simulink model "L21MSDsim"  (R2020a)
settings: Solver=FixedStepAuto  StartTime=0.0  StopTime=10  FixedStep=0.001  RelTol=1e-3
InitFcn:
  | L21MSDparameters;
values from neighbouring files (symbols this model uses):
  A = [0 1 ; -k/m -b/m]    [L21MSDparameters.m]
  B = [0 ; 1/m]    [L21MSDparameters.m]
  C = [1 0]    [L21MSDparameters.m]
  L = place(A',C',[-10 -20])'    [L21MSDparameters.m]
  x0 = [1; 0.5]    [L21MSDparameters.m]
  x0hat = [x0(1); 0]    [L21MSDparameters.m]
undefined symbols (not defined in the file or in its folder): LKB
libraries: simulink x1
settings Model: Creator=vcichella  LastModifiedBy=vcichella

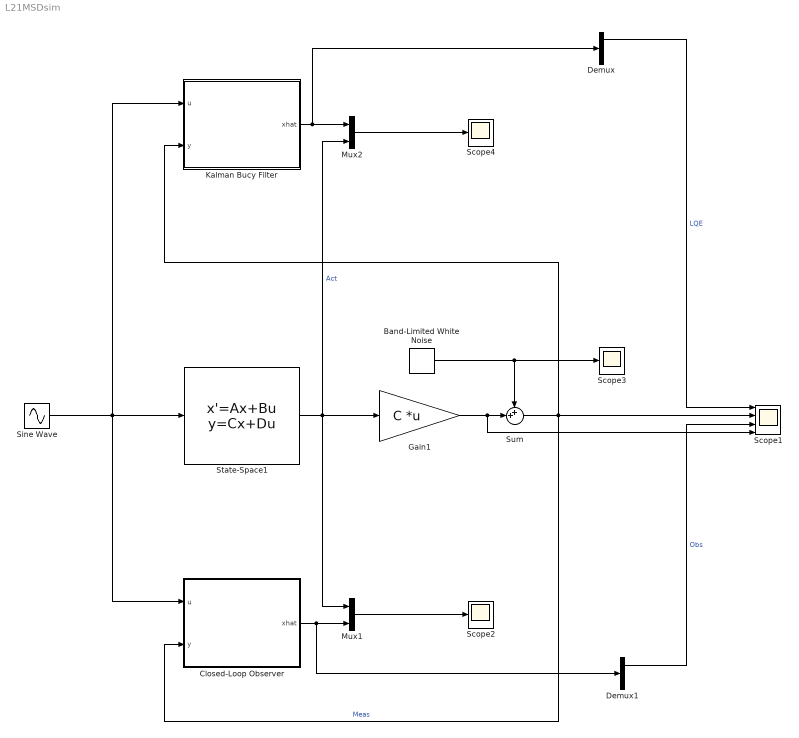
== system L21MSDsim ==
  Band-Limited White Noise : simulink/Sources/Band-Limited White Noise  Cov=[0.01]  Ts=0.01  seed=[23341]
  Closed-Loop Observer : Subsystem
  Demux : Demux  Outputs=2
  Demux1 : Demux  Outputs=2
  Gain1 : Gain  Gain=C  Multiplication=Matrix(K*u)
  Kalman Bucy Filter : Subsystem
  Mux1 : Mux  Inputs=2
  Mux2 : Mux  Inputs=2
  Scope1 : Scope  NumInputPorts=4
  Scope2 : Scope
  Scope3 : Scope
  Scope4 : Scope
  Sine Wave : Sin  Frequency=0.1  SampleTime=0
  State-Space1 : StateSpace  A=A  B=B  C=eye(size(A))  D=zeros(2,1)  InitialCondition=x0
  Sum : Sum  Inputs=++|
  wires:
  State-Space1/1 -> Mux2/2, Mux1/1, Gain1/1  "Act"
  Sine Wave/1 -> Kalman Bucy Filter/1(u), Closed-Loop Observer/1(u), State-Space1/1
  Closed-Loop Observer/1(xhat) -> Mux1/2, Demux1/1
  Mux1/1 -> Scope2/1
  Sum/1 -> Kalman Bucy Filter/2(y), Scope1/2, Closed-Loop Observer/2(y)  "Meas"
  Gain1/1 -> Scope1/4, Sum/2
  Band-Limited White Noise/1 -> Sum/1, Scope3/1
  Mux2/1 -> Scope4/1
  Kalman Bucy Filter/1(xhat) -> Mux2/1, Demux/1
  Demux1/1 -> Scope1/3  "Obs"
  Demux/1 -> Scope1/1  "LQE"

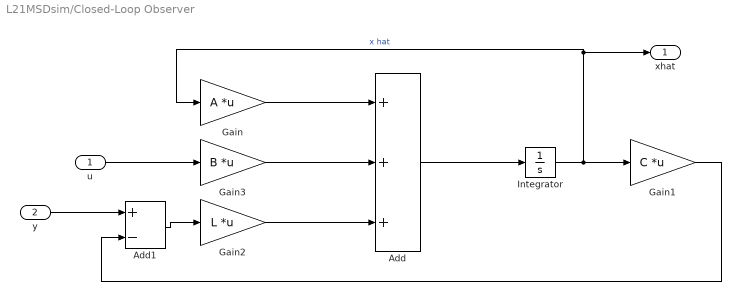
== system L21MSDsim/Closed-Loop Observer ==
  u : Inport
  y : Inport  Port=2
  Add : Sum  Inputs=+++
  Add1 : Sum  Inputs=+-
  Gain : Gain  Gain=A  Multiplication=Matrix(K*u)
  Gain1 : Gain  Gain=C  Multiplication=Matrix(K*u)
  Gain2 : Gain  Gain=L  Multiplication=Matrix(K*u)
  Gain3 : Gain  Gain=B  Multiplication=Matrix(K*u)
  Integrator : Integrator  InitialCondition=x0hat
  xhat : Outport
  wires:
  Integrator/1 -> xhat/1, Gain/1, Gain1/1  "x hat"
  Add/1 -> Integrator/1
  Gain/1 -> Add/1
  Gain1/1 -> Add1/2
  Add1/1 -> Gain2/1
  y/1 -> Add1/1
  Gain2/1 -> Add/3
  u/1 -> Gain3/1
  Gain3/1 -> Add/2

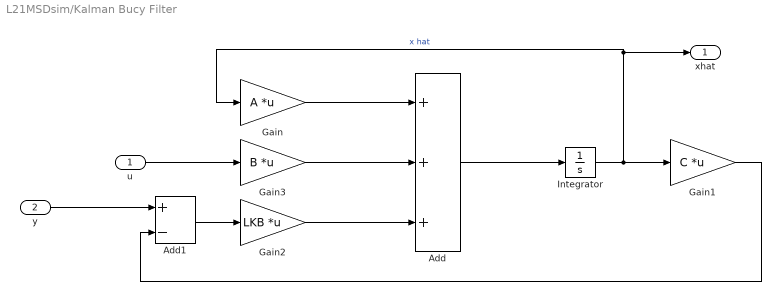
== system L21MSDsim/Kalman Bucy Filter ==
  u : Inport
  y : Inport  Port=2
  Add : Sum  Inputs=+++
  Add1 : Sum  Inputs=+-
  Gain : Gain  Gain=A  Multiplication=Matrix(K*u)
  Gain1 : Gain  Gain=C  Multiplication=Matrix(K*u)
  Gain2 : Gain  Gain=LKB  Multiplication=Matrix(K*u)
  Gain3 : Gain  Gain=B  Multiplication=Matrix(K*u)
  Integrator : Integrator  InitialCondition=x0hat
  xhat : Outport
  wires:
  Gain3/1 -> Add/2
  u/1 -> Gain3/1
  Gain2/1 -> Add/3
  y/1 -> Add1/1
  Add1/1 -> Gain2/1
  Gain1/1 -> Add1/2
  Gain/1 -> Add/1
  Add/1 -> Integrator/1
  Integrator/1 -> Gain1/1, Gain/1, xhat/1  "x hat"
